simulink model "maglev_control"  (Simulink 7.3)
settings: Solver=ode45  StartTime=0.0  StopTime=10.0  MaxStep=0.1  RelTol=1e-3
values from neighbouring files (symbols this model uses):
  h0 = 0.02    [MagnetLev.m]    (also in MagnetModel.m)
undefined symbols (not defined in the file or in its folder): den, num, v0
settings Model: Creator=sn00632  LastModifiedBy=sn00632

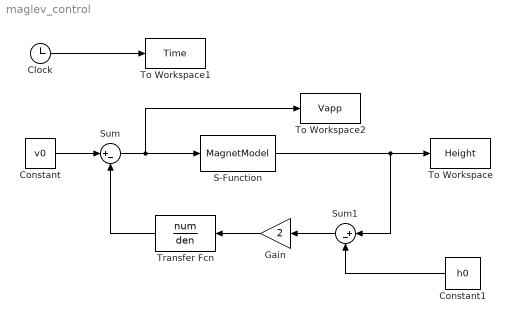
== system maglev_control ==
  Clock : Clock
      settings: Decimation=10
  Constant : Constant  Value=v0  OutDataType=fixdt(1, 16)  OutScaling=2^0
  Constant1 : Constant  Value=h0  OutDataType=fixdt(1, 16)  OutScaling=2^0
  Gain : Gain  Gain=2  ParameterDataType=fixdt(1, 16)  ParameterScaling=2^0  OutDataType=fixdt(1, 16)  OutScaling=2^0
  S-Function : S-Function  FunctionName=MagnetModel  EnableBusSupport=off
  Sum : Sum  Inputs=|+-  OutDataType=fixdt(1, 16)  OutScaling=2^0
  Sum1 : Sum  Inputs=|+-  OutDataType=fixdt(1, 16)  OutScaling=2^0
  To Workspace : ToWorkspace  VariableName=Height  SampleTime=-1  SaveFormat=Array
  To Workspace1 : ToWorkspace  VariableName=Time  SampleTime=-1  SaveFormat=Array
  To Workspace2 : ToWorkspace  VariableName=Vapp  SampleTime=-1  SaveFormat=Array
  Transfer Fcn : TransferFcn  Numerator=num  Denominator=den
  wires:
  Clock/1 -> To Workspace1/1
  Constant/1 -> Sum/1
  Sum/1 -> S-Function/1, To Workspace2/1
  Transfer Fcn/1 -> Sum/2
  Gain/1 -> Transfer Fcn/1
  Sum1/1 -> Gain/1
  Constant1/1 -> Sum1/2
  S-Function/1 -> To Workspace/1, Sum1/1
